simulink model "COP_Master"  (R2019a)
settings: Solver=FixedStepAuto  StartTime=0.0  StopTime=70  FixedStep=Ts  RelTol=1e-3  EnableMultiTasking=on
values from neighbouring files (symbols this model uses):
  f1_off = 0    [msstudy.m]    (also in pbase_l.m = nanmean(tsmovavg(Input3.data(1:40000,1),'s',1000,1)))
  f2_off = 0    [msstudy.m]    (also in pbase_l.m = nanmean(tsmovavg(Input3.data(1:40000,2),'s',1000,1)))
  f3_off = 0    [msstudy.m]    (also in pbase_l.m = nanmean(tsmovavg(Input3.data(1:40000,3),'s',1000,1)))
  f4_off = 0    [msstudy.m]    (also in pbase_l.m = nanmean(tsmovavg(Input3.data(1:40000,4),'s',1000,1)))
  f5_off = 0    [msstudy.m]    (also in pbase_l.m = nanmean(tsmovavg(Input3.data(1:40000,5),'s',1000,1)))
  f6_off = 0    [msstudy.m]    (also in pbase_l.m = nanmean(tsmovavg(Input3.data(1:40000,6),'s',1000,1)))
  f7_off = 0    [msstudy.m]    (also in pbase_l.m = nanmean(tsmovavg(Input3.data(1:40000,7),'s',1000,1)))
  f8_off = 0    [msstudy.m]    (also in pbase_l.m = nanmean(tsmovavg(Input3.data(1:40000,8),'s',1000,1)))
  kdp = str2double(get(handles.kdp,'String'))    [msstudy.m]
  kie = str2double(get(handles.kie,'String'))    [msstudy.m]
  maxtorquediff = 50    [msstudy.m]
  Ts = 0.0005    [msstudy.m]
  ttime = 2000*str2double(get(handles.ttime,'String'))    [msstudy.m]
  tweight = 50*0.01*weight    [msstudy.m]    (also in weightcalc.m = weight/2)
  visual = 1    [msstudy.m]
undefined symbols (not defined in the file or in its folder): Pull, up
libraries: speedgoatlib_IO183 x8, dspsigops x2, slrtlib x2, cstblocks x2
settings Model: TunableVars=kdp,kie,ttime  TunableVarsStorageClass=Auto,Auto,Auto  TunableVarsTypeQualifier=,,  Creator=vnalam  LastModifiedBy=vnalam
settings DataIOCC: LimitDataPoints=on  SaveFormat=StructureWithTime  ReturnWorkspaceOutputs=off
settings OptimizationCC: BlockReduction=off  OptimizeBlockIOStorage=off  BufferReuse=off  GlobalBufferReuse=off  ExpressionFolding=off  LocalBlockOutputs=off  LifeSpan=inf  OptimizeDataStoreBuffers=off  BusAssignmentInplaceUpdate=off
settings DebuggingCC: AllowSymbolicDim=off  SFUnexpectedBacktrackingDiag=warning  SFNoUnconditionalDefaultTransitionDiag=warning  SFExecutionAtInitializationDiag=none  ArithmeticOperatorsInVariantConditions=warning
settings HardwareCC: ProdBitPerPointer=32  ProdBitPerSizeT=32  ProdBitPerPtrDiffT=32  ProdLargestAtomicFloat=None  ProdWordSize=32  ProdLongLongMode=on  ProdHWDeviceType=Generic->32-bit x86 compatible
settings ModelReferenceCC: PropagateSignalLabelsOutOfModel=off
settings SFSimCC: SimUseLocalCustomCode=off
settings RTWCC: SystemTargetFile=slrt.tlc  TLCOptions=-axPCModelStackSizeKB=512  TemplateMakefile=slrt_default_tmf  Description=Simulink Real-Time  RTWUseLocalCustomCode=off  CodeExecutionProfiling=on  RTWCompilerOptimization=on
settings CodeAppCC: StateflowObjectComments=on
settings SimulinkRealTimeCC: PreserveStateflowLocalDataDimensions=off  RL32LogTETModifier=off  xPCConcurrentTasks=on
settings ConfigComp: CovMetricSettings=dw  CovHtmlReporting=on  CovSaveCumulativeToWorkspaceVar=on  CovSaveSingleToWorkspaceVar=on  CovExternalEMLEnable=off

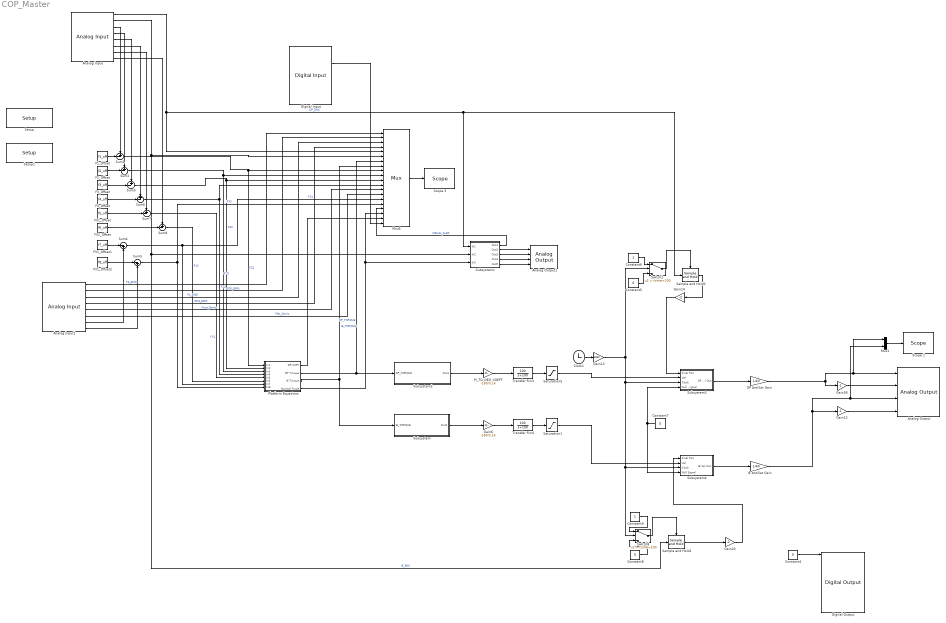
== system COP_Master ==
  Analog Input : speedgoatlib_IO183/Analog Input  Priority=0  parModuleId=1  parSampTime=Ts  parPciSlot=-1  parAdChannelLow=1  parAdChannelHigh=8
      settings: SourceProductName=Simulink Real-Time: Speedgoat Library
  Analog Input1 : speedgoatlib_IO183/Analog Input  Priority=0  parModuleId=2  parSampTime=Ts  parPciSlot=-1  parAdChannelLow=1  parAdChannelHigh=8
      settings: SourceProductName=Simulink Real-Time: Speedgoat Library
  Analog Output : speedgoatlib_IO183/Analog Output  parModuleId=1  parSampTime=-1  parDaSimult=on  parPciSlot=-1  parDaChannels=[1 2 3 4]  parDaInit=[0 0 0 0]  parDaReset=[0 0 0 0]
      settings: SourceProductName=Simulink Real-Time: Speedgoat Library
  Analog Output1 : speedgoatlib_IO183/Analog Output  parModuleId=2  parSampTime=-1  parDaSimult=on  parPciSlot=-1  parDaChannels=[1 2 3 4]  parDaInit=[0 0 0 0]  parDaReset=[0 0 0 0]
      settings: SourceProductName=Simulink Real-Time: Speedgoat Library
  Clock1 : Clock
  Constant{4..5,7..8} (4 alike) : Constant  Value=0  SampleTime=Ts
  Constant6 : Constant  SampleTime=Ts
  Constant9 : Constant  SampleTime=Ts
  DP AntiSat Gain : Gain  Gain=1/40
  Digital Input : speedgoatlib_IO183/Digital Input  parModuleId=2  parSampTime=Ts  parPciSlot=-1  parDiChannels=[9 10 11 12 13 14 15 16]
      settings: SourceProductName=Simulink Real-Time: Speedgoat Library
  Digital Output : speedgoatlib_IO183/Digital Output  parModuleId=2  parSampTime=Ts  parPciSlot=-1  parDoChannels=[1 2 3 4 5 6 7 8]  parDoInit=[0 0 0 0 0 0 0 0]  parDoReset=[1 1 1 1 1 1 1 1]
      settings: SourceProductName=Simulink Real-Time: Speedgoat Library
  F1_Offset : Constant  Value=f1_off  SampleTime=Ts
  F2_Offset : Constant  Value=f2_off  SampleTime=Ts
  F3_Offset : Constant  Value=f3_off  SampleTime=Ts
  F4_Offset : Constant  Value=f4_off  SampleTime=Ts
  FX1_Offset : Constant  Value=f5_off  SampleTime=Ts
  FX1_Offset1 : Constant  Value=f7_off  SampleTime=Ts
  FX1_Offset2 : Constant  Value=f8_off  SampleTime=Ts
  FX2_Offset : Constant  Value=f6_off  SampleTime=Ts
  Gain12 : Gain  Gain=-1
  Gain13 : Gain  Gain=2000
  Gain14 : Gain  Gain=-2
  Gain20 : Gain  Gain=-2
  Gain36 : Gain  Gain=-1
  Gain6 : Gain  Gain=-180/3.14
  IE AntiSat Gain : Gain  Gain=1/40
  Mux1 : Mux  Inputs=2
  Mux6 : Mux  Inputs=20
      settings: DisplayOption=signals
  PI_TO_DEG_COEFF : Gain  Gain=-180/3.14
  Platform Equations : Subsystem
  Sample and Hold1 : dspsigops/Sample and Hold  trig=Rising edge  initCond=0  latchinput=off
  Sample and Hold2 : dspsigops/Sample and Hold  trig=Rising edge  initCond=0  latchinput=off
  Saturation1 : Saturate  UpperLimit=100  LowerLimit=-100
  Saturation5 : Saturate  UpperLimit=100  LowerLimit=-100
  Scope 1 : slrtlib/Displays and Logging/Scope   scopeno=2  scopetype=Target  autostart=on  viewmode=Graphical sliding  formatstr='%15.6f'  grid=on  ylimits=[0,0]  nosamples=10000  noprepostsamples=0  interleave=1  triggermode=FreeRun  triggersignal=1  trigsignalfromport=off  triggerlevel=0.0  triggerslope=Either  triggerscope=1  triggersample=0  filename=tot303.dat  mode=Lazy  writesize=512  autorestart=off  dynamicfilemode=off  maxwritefilesize=512*1024^2
  Scope 3 : slrtlib/Displays and Logging/Scope   scopeno=3  scopetype=File  autostart=on  viewmode=Graphical redraw  formatstr='%15.6f'  grid=on  ylimits=[0,0]  nosamples=1000000  noprepostsamples=0  interleave=1  triggermode=FreeRun  triggersignal=1  trigsignalfromport=off  triggerlevel=0.0  triggerslope=Either  triggerscope=1  triggersample=0  filename=COP_DEF.dat  mode=Commit  writesize=1024  autorestart=off  dynamicfilemode=off  maxwritefilesize=512*1024^2
  Setup : speedgoatlib_IO183/Setup  parModuleId=1  parPciSlot=-1  parDaSimult=on  parAdCoupling=Single Ended  parAdRange=+-10V  parAdChannelLow=1  parAdChannelHigh=8  parDaChannels=[1:4]  parDaRange=0..5V  parDaInit=[0]  parDaReset=[0]  parDoChannels=[1:8]  parDoInit=[0]  parDoReset=[1]  parDiChannels=[9:16]  parIOPullReferenceFront=Pull-up (3.3V)  parIOPullReferenceRear=Pull-up (3.3V)
      settings: SourceProductName=Simulink Real-Time: Speedgoat Library
  Setup1 : speedgoatlib_IO183/Setup  parModuleId=2  parPciSlot=-1  parDaSimult=on  parAdCoupling=Single Ended  parAdRange=+-10V  parAdChannelLow=1  parAdChannelHigh=8  parDaChannels=[1:4]  parDaRange=0..5V  parDaInit=[0]  parDaReset=[0]  parDoChannels=[1:8]  parDoInit=[0]  parDoReset=[1]  parDiChannels=[9:16]  parIOPullReferenceFront=Pull-up (3.3V)  parIOPullReferenceRear=Pull-up (3.3V)
      settings: SourceProductName=Simulink Real-Time: Speedgoat Library
  Subsystem : Subsystem
  Subsystem1 : Subsystem
  Subsystem2 : Subsystem
  Subsystem3 : Subsystem
  Subsystem4 : Subsystem
  Sum{1..3,6..8} (6 alike) : Sum  Inputs=+-|
  Sum4 : Sum  Inputs=|-+
  Sum5 : Sum  Inputs=|-+
  Switch2 : Switch  Criteria=u2 > Threshold  Threshold=ttime+200
  Switch8 : Switch  Criteria=u2 > Threshold  Threshold=ttime+200
  Transfer Fcn3 : TransferFcn  Numerator=[100]  Denominator=[1 100]
  Transfer Fcn4 : TransferFcn  Numerator=[100]  Denominator=[1 100]
  wires:
  Mux6/1 -> Scope 3/1
  Sum1/1 -> Platform Equations/1(In1), Mux6/9  "FZ1"
  Sum2/1 -> Platform Equations/3(In3), Mux6/10  "FZ2"
  Sum3/1 -> Mux6/11, Platform Equations/2(In2)  "FZ3"
  Sum6/1 -> Mux6/12, Platform Equations/4(In4)  "FZ4"
  Analog Input1/2 -> Mux6/2  "SOL_EMG"
  Analog Input1/3 -> Mux6/3  "PL_EMG"
  Analog Input1/7 -> Sum4/2
  Analog Input1/8 -> Sum5/2
  Analog Input1/1 -> Mux6/1  "TA_EMG"
  DP AntiSat Gain/1 -> Gain36/1, Analog Output/1, Mux1/1
  Analog Input1/5 -> Mux6/13  "Foot_Gonio"
  Analog Input1/4 -> Mux6/4  "GCA_EMG"
  Analog Input/3 -> Sum1/1
  Analog Input/4 -> Sum2/1
  Analog Input/5 -> Sum3/1
  Analog Input/6 -> Sum6/1
  F1_Offset/1 -> Sum1/2
  F2_Offset/1 -> Sum2/2
  F3_Offset/1 -> Sum3/2
  F4_Offset/1 -> Sum6/2
  Analog Input/7 -> Sum7/1
  FX1_Offset/1 -> Sum7/2
  Analog Input/8 -> Sum8/1
  FX2_Offset/1 -> Sum8/2
  PI_TO_DEG_COEFF/1 -> Transfer Fcn3/1
  Subsystem2/1(Out1) -> PI_TO_DEG_COEFF/1
  Transfer Fcn3/1 -> Saturation5/1
  Gain36/1 -> Analog Output/2
  Analog Input1/6 -> Mux6/14  "Plat_Gonio"
  Transfer Fcn4/1 -> Saturation1/1
  Gain6/1 -> Transfer Fcn4/1
  Gain12/1 -> Analog Output/4
  IE AntiSat Gain/1 -> Analog Output/3, Mux1/2, Gain12/1
  Mux1/1 -> Scope 1/1
  Clock1/1 -> Gain13/1
  Constant7/1 -> Subsystem4/4(Null Signal), Subsystem3/4(Null Signal)
  Switch2/1 -> Sample and Hold2/Trigger
  Analog Input/1 -> Sample and Hold2/1, Subsystem1/1(In1), Mux6/5  "DP_ENC"
  Sample and Hold2/1 -> Gain14/1
  Constant5/1 -> Switch2/3
  Constant6/1 -> Switch2/1
  Constant8/1 -> Switch8/3
  Gain13/1 -> Switch8/2, Subsystem4/3(Clock), Subsystem3/3(Clock), Switch2/2
  Constant9/1 -> Switch8/1
  Sample and Hold1/1 -> Gain20/1
  Analog Input/2 -> Sample and Hold1/1, Subsystem1/2(In2), Mux6/6  "IE_ENC"
  Switch8/1 -> Sample and Hold1/Trigger
  Constant4/1 -> Digital Output/1
  Platform Equations/4(Normal Force) -> Mux6/18, Subsystem1/3(In3)
  Platform Equations/2(DP Torque) -> Subsystem2/1(DP_TORQUE), Mux6/7  "DP_TORQUE"
  Platform Equations/3(IE Torque) -> Subsystem/1(IE_TORQUE), Mux6/8  "IE_TORQUE"
  Sum7/1 -> Platform Equations/5(In5)  "FX1"
  Sum8/1 -> Platform Equations/6(In6)  "FX2"
  Platform Equations/1(DP COP?) -> Mux6/19
  Subsystem1/1(Out1) -> Mux6/17  "VISUAL_FLAG"
  Subsystem1/2(Out2) -> Analog Output1/1
  Subsystem1/3(Out3) -> Analog Output1/2
  Subsystem1/4(Out4) -> Analog Output1/3
  Subsystem1/5(Out5) -> Analog Output1/4
  Saturation1/1 -> Subsystem4/2(Vel)
  Gain20/1 -> Subsystem4/1(Final Pos)
  Subsystem4/1(IE Vel Out) -> IE AntiSat Gain/1
  Gain14/1 -> Subsystem3/1(Final Pos)
  Saturation5/1 -> Subsystem3/2(Vel)
  Subsystem3/1(DP Vel Out) -> DP AntiSat Gain/1
  FX1_Offset1/1 -> Sum4/1
  FX1_Offset2/1 -> Sum5/1
  Sum4/1 -> Mux6/15, Platform Equations/7(In7)  "FX1"
  Sum5/1 -> Platform Equations/8(In8), Mux6/16  "FX2"
  Subsystem/1(Out1) -> Gain6/1
  Digital Input/3 -> Mux6/20

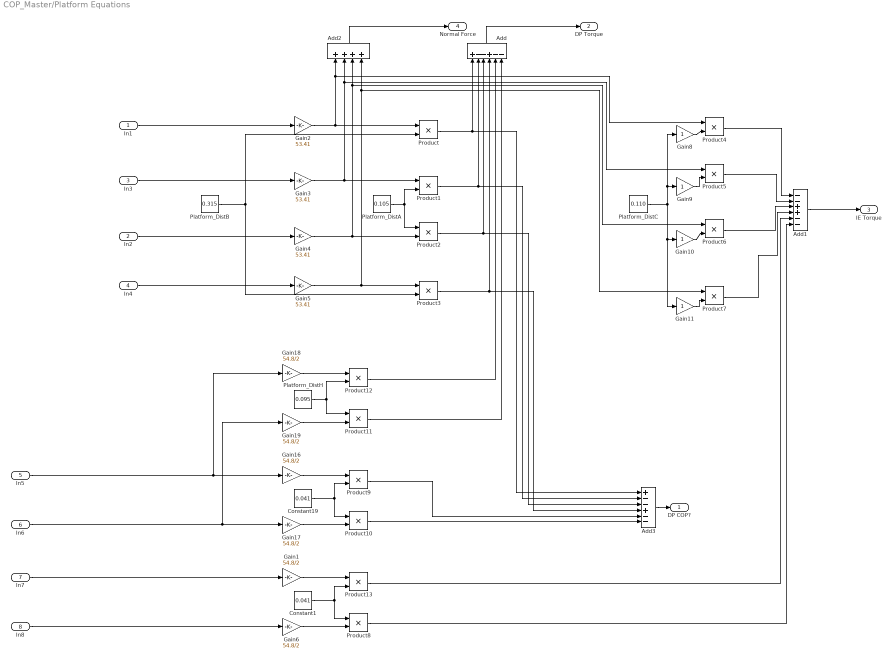
== system COP_Master/Platform Equations ==
  In1 : Inport
  In2 : Inport  Port=2
  In3 : Inport  Port=3
  In4 : Inport  Port=4
  In5 : Inport  Port=5
  In6 : Inport  Port=6
  In7 : Inport  Port=7
  In8 : Inport  Port=8
  Add : Sum  Inputs=+--+--
  Add1 : Sum  Inputs=--++--
  Add2 : Sum  Inputs=++++
  Add3 : Sum  Inputs=+--+--
  Constant1 : Constant  Value=0.041  SampleTime=-1
  Constant19 : Constant  Value=0.041  SampleTime=-1
  Gain{1,6,16..19} (6 alike) : Gain  Gain=54.8/2
  Gain{8..11} (4 alike) : Gain
  Gain{2..5} (4 alike) : Gain  Gain=53.41
  Platform_DistA : Constant  Value=0.105  SampleTime=-1
  Platform_DistB : Constant  Value=0.315  SampleTime=-1
  Platform_DistC : Constant  Value=0.110  SampleTime=-1
  Platform_DistH : Constant  Value=0.095  SampleTime=-1
  Product{,1..13} (14 alike) : Product
  DP COP? : Outport
  DP Torque : Outport  Port=2
  IE Torque : Outport  Port=3
  Normal Force : Outport  Port=4
  wires:
  Product6/1 -> Add1/3
  Gain3/1 -> Product5/1, Add2/2, Product1/1
  Product9/1 -> Add3/5
  Product10/1 -> Add3/6
  Product/1 -> Add/1, Add3/1
  Add1/1 -> IE Torque/1
  Add2/1 -> Normal Force/1
  Platform_DistA/1 -> Product2/1, Product1/2
  Platform_DistH/1 -> Product11/1, Product12/2
  Gain9/1 -> Product5/2
  Gain5/1 -> Product3/1, Product7/1, Add2/4
  In5/1 -> Gain16/1, Gain18/1
  Platform_DistC/1 -> Gain8/1, Gain9/1, Gain11/1, Gain10/1
  Gain2/1 -> Product/1, Product4/1, Add2/1
  Gain18/1 -> Product12/1
  Gain10/1 -> Product6/2
  Product2/1 -> Add3/3, Add/3
  Add/1 -> DP Torque/1
  Platform_DistB/1 -> Product3/2, Product/2
  In6/1 -> Gain17/1, Gain19/1
  In3/1 -> Gain3/1
  Product4/1 -> Add1/1
  Product3/1 -> Add3/4, Add/4
  Gain11/1 -> Product7/2
  Gain4/1 -> Product2/2, Product6/1, Add2/3
  Product11/1 -> Add/6
  Product12/1 -> Add/5
  Product5/1 -> Add1/2
  In1/1 -> Gain2/1
  Product1/1 -> Add/2, Add3/2
  Add3/1 -> DP COP?/1
  Gain8/1 -> Product4/2
  Gain16/1 -> Product9/1
  Product7/1 -> Add1/4
  In2/1 -> Gain4/1
  In4/1 -> Gain5/1
  Gain17/1 -> Product10/2
  Constant19/1 -> Product9/2, Product10/1
  Gain19/1 -> Product11/2
  Constant1/1 -> Product13/2, Product8/1
  Gain6/1 -> Product8/2
  In7/1 -> Gain1/1
  Gain1/1 -> Product13/1
  In8/1 -> Gain6/1
  Product13/1 -> Add1/5
  Product8/1 -> Add1/6

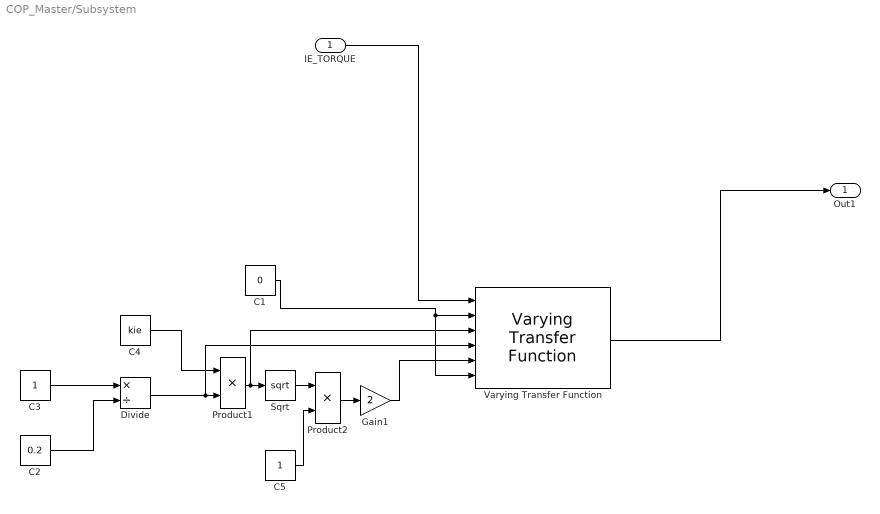
== system COP_Master/Subsystem ==
  IE_TORQUE : Inport
  C1 : Constant  Value=0  SampleTime=Ts
  C2 : Constant  Value=0.2  SampleTime=Ts
  C3 : Constant  SampleTime=Ts
  C4 : Constant  Value=kie  SampleTime=Ts
  C5 : Constant  SampleTime=Ts
  Divide : Product  Inputs=*/
  Gain1 : Gain  Gain=2
  Product1 : Product
  Product2 : Product
  Sqrt : Sqrt  SaturateOnIntegerOverflow=on
  Varying Transfer Function : cstblocks/Linear Parameter Varying/Varying Transfer Function  N=2
      settings: SourceProductName=Control System Toolbox
  Out1 : Outport
  wires:
  Gain1/1 -> Varying Transfer Function/5
  C3/1 -> Divide/1
  C5/1 -> Product2/2
  C2/1 -> Divide/2
  Divide/1 -> Varying Transfer Function/4, Product1/2
  Product1/1 -> Varying Transfer Function/3, Sqrt/1
  C4/1 -> Product1/1
  Sqrt/1 -> Product2/1
  C1/1 -> Varying Transfer Function/6, Varying Transfer Function/2
  Product2/1 -> Gain1/1
  IE_TORQUE/1 -> Varying Transfer Function/1
  Varying Transfer Function/1 -> Out1/1

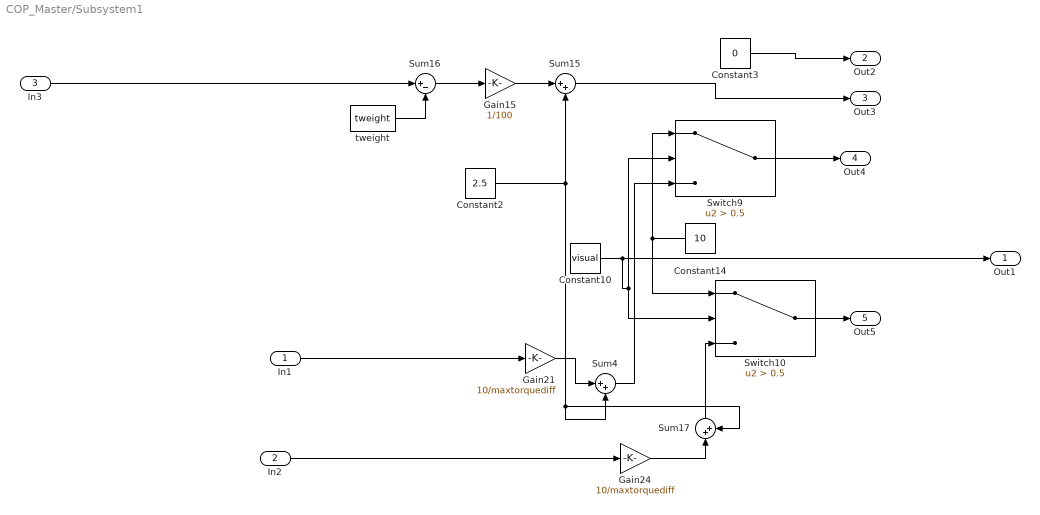
== system COP_Master/Subsystem1 ==
  In1 : Inport
  In2 : Inport  Port=2
  In3 : Inport  Port=3
  Constant10 : Constant  Value=visual  SampleTime=Ts
  Constant14 : Constant  Value=10  SampleTime=Ts
  Constant2 : Constant  Value=2.5  SampleTime=Ts
  Constant3 : Constant  Value=0  SampleTime=Ts
  Gain15 : Gain  Gain=1/100
  Gain21 : Gain  Gain=10/maxtorquediff
  Gain24 : Gain  Gain=10/maxtorquediff
  Sum15 : Sum  Inputs=|++
  Sum16 : Sum  Inputs=|+-
  Sum17 : Sum  Inputs=|++
  Sum4 : Sum  Inputs=|++
  Switch10 : Switch  Criteria=u2 > Threshold  Threshold=0.5
  Switch9 : Switch  Criteria=u2 > Threshold  Threshold=0.5
  tweight : Constant  Value=tweight  SampleTime=Ts
  Out1 : Outport
  Out2 : Outport  Port=2
  Out3 : Outport  Port=3
  Out4 : Outport  Port=4
  Out5 : Outport  Port=5
  wires:
  Constant14/1 -> Switch10/1, Switch9/1
  Gain24/1 -> Sum17/1
  Sum16/1 -> Gain15/1
  Sum15/1 -> Out3/1
  Gain15/1 -> Sum15/1
  Gain21/1 -> Sum4/1
  Sum4/1 -> Switch9/3
  Constant10/1 -> Switch10/2, Switch9/2, Out1/1
  Sum17/1 -> Switch10/3
  tweight/1 -> Sum16/2
  Constant2/1 -> Sum15/2, Sum4/2, Sum17/2
  In3/1 -> Sum16/1
  In2/1 -> Gain24/1
  Switch10/1 -> Out5/1
  Switch9/1 -> Out4/1
  Constant3/1 -> Out2/1
  In1/1 -> Gain21/1

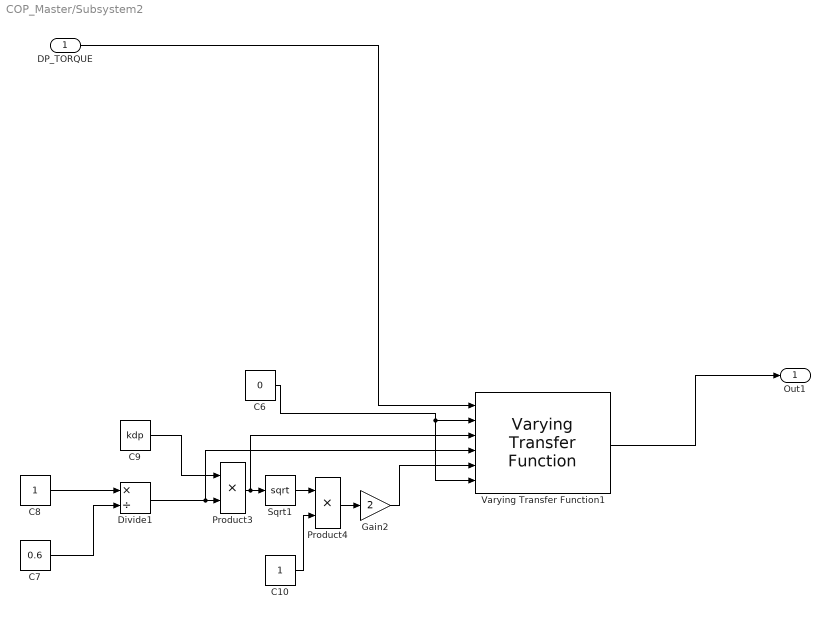
== system COP_Master/Subsystem2 ==
  DP_TORQUE : Inport
  C10 : Constant  SampleTime=Ts
  C6 : Constant  Value=0  SampleTime=Ts
  C7 : Constant  Value=0.6  SampleTime=Ts
  C8 : Constant  SampleTime=Ts
  C9 : Constant  Value=kdp  SampleTime=Ts
  Divide1 : Product  Inputs=*/
  Gain2 : Gain  Gain=2
  Product3 : Product
  Product4 : Product
  Sqrt1 : Sqrt  SaturateOnIntegerOverflow=on
  Varying Transfer Function1 : cstblocks/Linear Parameter Varying/Varying Transfer Function  N=2
      settings: SourceProductName=Control System Toolbox
  Out1 : Outport
  wires:
  C6/1 -> Varying Transfer Function1/6, Varying Transfer Function1/2
  Product3/1 -> Varying Transfer Function1/3, Sqrt1/1
  Product4/1 -> Gain2/1
  C7/1 -> Divide1/2
  Divide1/1 -> Varying Transfer Function1/4, Product3/2
  C9/1 -> Product3/1
  Gain2/1 -> Varying Transfer Function1/5
  Sqrt1/1 -> Product4/1
  C10/1 -> Product4/2
  C8/1 -> Divide1/1
  Varying Transfer Function1/1 -> Out1/1
  DP_TORQUE/1 -> Varying Transfer Function1/1

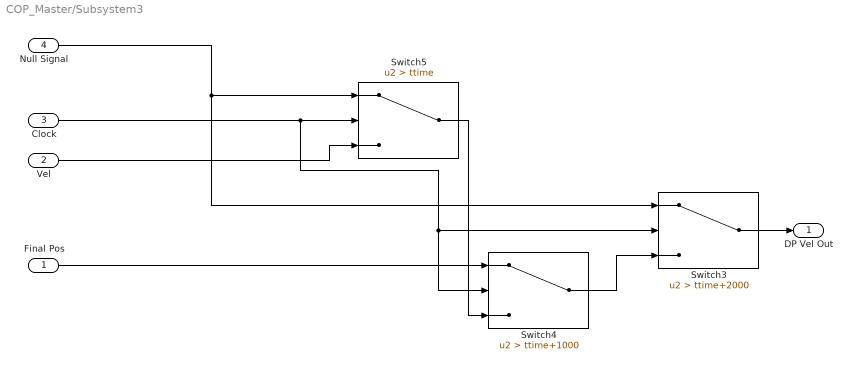
== system COP_Master/Subsystem3 ==
  Final Pos : Inport
  Vel : Inport  Port=2
  Clock : Inport  Port=3
  Null Signal : Inport  Port=4
  Switch3 : Switch  Criteria=u2 > Threshold  Threshold=ttime+2000
  Switch4 : Switch  Criteria=u2 > Threshold  Threshold=ttime+1000
  Switch5 : Switch  Criteria=u2 > Threshold  Threshold=ttime
  DP Vel Out : Outport
  wires:
  Vel/1 -> Switch5/3
  Clock/1 -> Switch3/2, Switch4/2, Switch5/2
  Final Pos/1 -> Switch4/1
  Null Signal/1 -> Switch5/1, Switch3/1
  Switch4/1 -> Switch3/3
  Switch3/1 -> DP Vel Out/1
  Switch5/1 -> Switch4/3

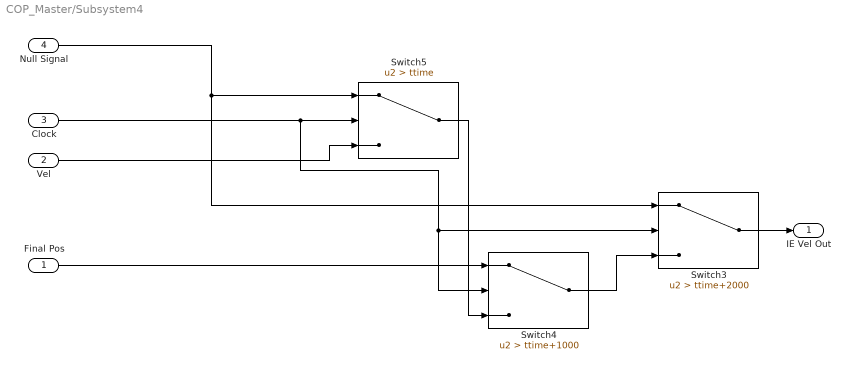
== system COP_Master/Subsystem4 ==
  Final Pos : Inport
  Vel : Inport  Port=2
  Clock : Inport  Port=3
  Null Signal : Inport  Port=4
  Switch3 : Switch  Criteria=u2 > Threshold  Threshold=ttime+2000
  Switch4 : Switch  Criteria=u2 > Threshold  Threshold=ttime+1000
  Switch5 : Switch  Criteria=u2 > Threshold  Threshold=ttime
  IE Vel Out : Outport
  wires:
  Vel/1 -> Switch5/3
  Clock/1 -> Switch3/2, Switch4/2, Switch5/2
  Final Pos/1 -> Switch4/1
  Null Signal/1 -> Switch5/1, Switch3/1
  Switch4/1 -> Switch3/3
  Switch3/1 -> IE Vel Out/1
  Switch5/1 -> Switch4/3
